simulink model "TransitionTypeHandler"  (R2016b)
settings: Solver=VariableStepAuto  StartTime=0.0  StopTime=10.0  RelTol=1e-3
settings Model: Creator=march  LastModifiedBy=march

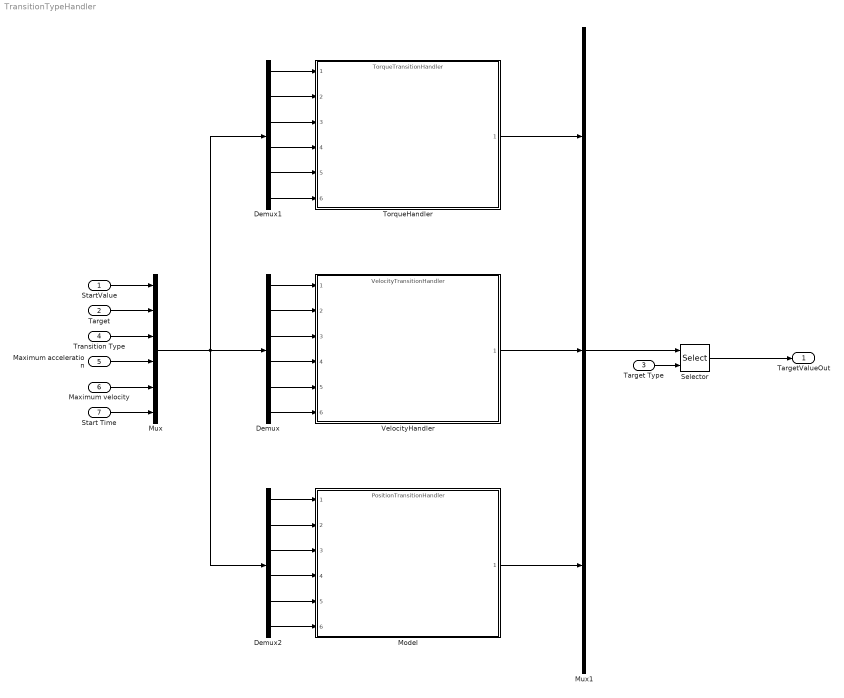
== system TransitionTypeHandler ==
  StartValue : Inport
  Target : Inport  Port=2
  Target Type : Inport  Port=3
  Transition Type : Inport  Port=4
  Maximum acceleration : Inport  Port=5
  Maximum velocity : Inport  Port=6
  Start Time : Inport  Port=7
  Demux : Demux  Outputs=6
  Demux1 : Demux  Outputs=6
  Demux2 : Demux  Outputs=6
  Model : ModelReference  ModelNameDialog=PositionTransitionHandler  SimulationMode=Normal  ModelReferenceVersion=1.2
  Mux : Mux  Inputs=6
  Mux1 : Mux  Inputs=3
  Selector : Selector  InputPortWidth=3  IndexOptions=Index vector (port)  Indices=[1 3]  OutputSizes=1
  TorqueHandler : ModelReference  ModelNameDialog=TorqueTransitionHandler  SimulationMode=Normal  ModelReferenceVersion=1.3
  VelocityHandler : ModelReference  ModelNameDialog=VelocityTransitionHandler  SimulationMode=Normal  ModelReferenceVersion=1.1
  TargetValueOut : Outport
  wires:
  Start Time/1 -> Mux/6
  StartValue/1 -> Mux/1
  Target/1 -> Mux/2
  Maximum acceleration/1 -> Mux/4
  Maximum velocity/1 -> Mux/5
  Transition Type/1 -> Mux/3
  Demux/1 -> VelocityHandler/1
  Demux/4 -> VelocityHandler/4
  Demux/3 -> VelocityHandler/3
  Demux/6 -> VelocityHandler/6
  Demux/5 -> VelocityHandler/5
  Demux/2 -> VelocityHandler/2
  Mux/1 -> Demux2/1, Demux1/1, Demux/1
  Demux1/2 -> TorqueHandler/2
  Demux1/4 -> TorqueHandler/4
  Demux1/5 -> TorqueHandler/5
  Demux1/6 -> TorqueHandler/6
  Demux1/1 -> TorqueHandler/1
  Demux1/3 -> TorqueHandler/3
  Demux2/3 -> Model/3
  Demux2/1 -> Model/1
  Demux2/4 -> Model/4
  Demux2/5 -> Model/5
  Demux2/2 -> Model/2
  Demux2/6 -> Model/6
  VelocityHandler/1 -> Mux1/2
  TorqueHandler/1 -> Mux1/1
  Model/1 -> Mux1/3
  Target Type/1 -> Selector/2
  Mux1/1 -> Selector/1
  Selector/1 -> TargetValueOut/1
